simulink model "week2_3"  (R2020b)
settings: Solver=VariableStepAuto  StartTime=0.0  StopTime=10.0  RelTol=1e-3
settings Model: Creator=Lenovo  LastModifiedBy=Lenovo

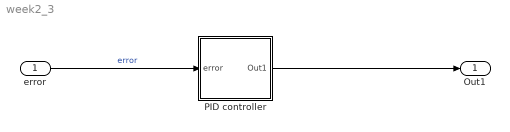
== system week2_3 ==
  error : Inport  OutDataTypeStr=double  PortDimensions=1  SampleTime=0
  PID controller : Subsystem
  Out1 : Outport  OutDataTypeStr=double  PortDimensions=1  SampleTime=0
  wires:
  error/1 -> PID controller/1(error)  "error"
  PID controller/1(Out1) -> Out1/1

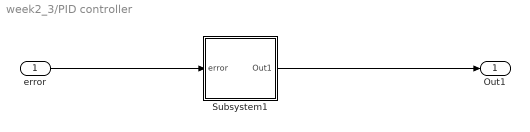
== system week2_3/PID controller ==
  error : Inport  OutDataTypeStr=double  PortDimensions=1  SampleTime=0
  Subsystem1 : Subsystem
  Out1 : Outport  OutDataTypeStr=double  PortDimensions=1  SampleTime=0
  wires:
  Subsystem1/1(Out1) -> Out1/1
  error/1 -> Subsystem1/1(error)

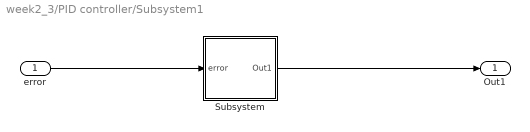
== system week2_3/PID controller/Subsystem1 ==
  error : Inport
  Subsystem : Subsystem
  Out1 : Outport
  wires:
  error/1 -> Subsystem/1(error)
  Subsystem/1(Out1) -> Out1/1

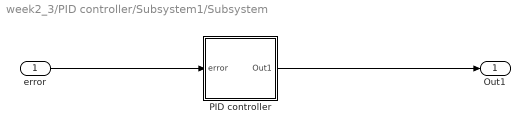
== system week2_3/PID controller/Subsystem1/Subsystem ==
  error : Inport  OutDataTypeStr=double  PortDimensions=1  SampleTime=0
  PID controller : Subsystem  TreatAsAtomicUnit=on
  Out1 : Outport  OutDataTypeStr=double  PortDimensions=1  SampleTime=0
  wires:
  error/1 -> PID controller/1(error)
  PID controller/1(Out1) -> Out1/1

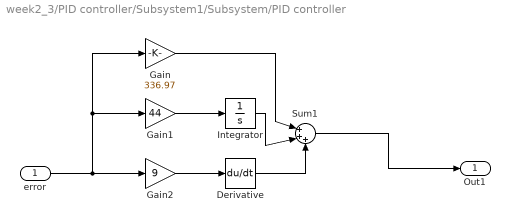
== system week2_3/PID controller/Subsystem1/Subsystem/PID controller ==
  error : Inport
  Derivative : Derivative
  Gain : Gain  Gain=336.97
  Gain1 : Gain  Gain=44
  Gain2 : Gain  Gain=9
  Integrator : Integrator
  Sum1 : Sum  Inputs=|+++
  Out1 : Outport
  wires:
  Gain1/1 -> Integrator/1
  Gain/1 -> Sum1/1
  Sum1/1 -> Out1/1
  error/1 -> Gain2/1, Gain1/1, Gain/1
  Derivative/1 -> Sum1/3
  Gain2/1 -> Derivative/1
  Integrator/1 -> Sum1/2
